simulink model "lab5_simulink"  (R2019a)
settings: Solver=VariableStepAuto  StartTime=0.0  StopTime=10.0  RelTol=1e-3
values from neighbouring files (symbols this model uses):
  b = 0.1    [variables_lab5.m]
  J = 0.01    [variables_lab5.m]
  K = 0.01    [variables_lab5.m]
  L = 0.5    [variables_lab5.m]
  R = 1    [variables_lab5.m]
settings Model: Creator=abc  LastModifiedBy=abc

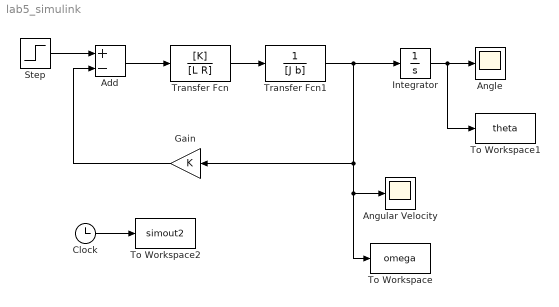
== system lab5_simulink ==
  Add : Sum  Inputs=+-
  Angle : Scope
  "Angular Velocity " : Scope
  Clock : Clock
  Gain : Gain  Gain=K
  Integrator : Integrator
  Step : Step  Time=0.1  After=0.02  SampleTime=0
  To Workspace : ToWorkspace  VariableName=omega  SaveFormat=Timeseries  SampleTime=-1
  To Workspace1 : ToWorkspace  VariableName=theta  SaveFormat=Timeseries  SampleTime=-1
  To Workspace2 : ToWorkspace  VariableName=simout2  SaveFormat=Timeseries  SampleTime=-1
  Transfer Fcn : TransferFcn  Numerator=[K]  Denominator=[L R]
  Transfer Fcn1 : TransferFcn  Denominator=[J b]
  wires:
  Transfer Fcn/1 -> Transfer Fcn1/1
  Gain/1 -> Add/2
  Step/1 -> Add/1
  Add/1 -> Transfer Fcn/1
  Integrator/1 -> To Workspace1/1, Angle/1
  Transfer Fcn1/1 -> To Workspace/1, "Angular Velocity "/1, Gain/1, Integrator/1
  Clock/1 -> To Workspace2/1
